simulink model "ModeloSimulador"  (R2020a)
settings: Solver=ode5  StartTime=0.0  StopTime=10.0  FixedStep=0.0001  RelTol=1e-3
values from neighbouring files (symbols this model uses):
  Bm = 0.008    [definirParametros.m]    (also in definirParametrosMotorElectroCraftDP300.m; definirParametrosMotorElectroCraftDPP728V120.m = Jm/tm; definirParametrosMotorElectroCraftDPP728V120_Optimizador.m = Jm/tm; definirParametrosMotorElectroCraftDPP728V120_v2.m = Jm/tm)
  dm = 0.3    [definirParametros.m]    (also in definirParametrosMotorElectroCraftDP300.m; definirParametrosMotorElectroCraftDPP728V120.m; definirParametrosMotorElectroCraftDPP728V120_Optimizador.m = 0.550061; definirParametrosMotorElectroCraftDPP728V120_v2.m = 0.550061)
  dmc = 0.5    [definirParametros.m]    (also in definirParametrosMotorElectroCraftDP300.m; definirParametrosMotorElectroCraftDPP728V120.m; definirParametrosMotorElectroCraftDPP728V120_Optimizador.m = 1.06911; definirParametrosMotorElectroCraftDPP728V120_v2.m = 1.06911)
  g = 9.8    [definirParametros.m]    (also in definirParametrosMotorElectroCraftDP300.m; definirParametrosMotorElectroCraftDPP728V120.m; definirParametrosMotorElectroCraftDPP728V120_Optimizador.m; definirParametrosMotorElectroCraftDPP728V120_v2.m)
  Jm = gramsCM2ToKgMeters2(12358.5)    [definirParametrosMotorElectroCraftDPP728V120.m]    (also in definirParametrosMotorElectroCraftDPP728V120_Optimizador.m; definirParametrosMotorElectroCraftDPP728V120_v2.m; definirParametrosMotorElectroCraftDPP728V120_v3.m; definirParametrosMotorElectroCraftRP34M221V90.m = gramsCM2ToKgMeters2(2718.9))
  Kb = 0.6    [definirParametros.m]    (also in definirParametrosMotorElectroCraftDP300.m = VoltagePerKRPMToVoltagePerHertz(12.3); definirParametrosMotorElectroCraftDPP728V120.m = VoltagePerKRPMToVoltagePerRadS(64.9); definirParametrosMotorElectroCraftDPP728V120_Optimizador.m = VoltagePerKRPMToVoltagePerRadS(64.9); definirParametrosMotorElectroCraftDPP728V120_v2.m = VoltagePerKRPMToVoltagePerRadS(64.9))
  Kt = 0.7274    [definirParametros.m]    (also in definirParametrosMotorElectroCraftDP300.m = newtonCMToNewtonM(11.722); definirParametrosMotorElectroCraftDPP728V120.m = newtonCMToNewtonM(62); definirParametrosMotorElectroCraftDPP728V120_Optimizador.m = newtonCMToNewtonM(62); definirParametrosMotorElectroCraftDPP728V120_v2.m = newtonCMToNewtonM(62))
  Lm = 4.3/1000    (= 0.0043)    [definirParametrosMotorElectroCraftDPP728V120.m]    (also in definirParametrosMotorElectroCraftDPP728V120_Optimizador.m; definirParametrosMotorElectroCraftDPP728V120_v2.m; definirParametrosMotorElectroCraftDPP728V120_v3.m; definirParametrosMotorElectroCraftDPP728V60.m = 0.0015)
  Mc = 200    [definirParametros.m]    (also in definirParametrosMotorElectroCraftDP300.m; definirParametrosMotorElectroCraftDPP728V120.m; definirParametrosMotorElectroCraftDPP728V120_Optimizador.m = 144.6; definirParametrosMotorElectroCraftDPP728V120_v2.m = 144.6)
  Mm = 100    [definirParametros.m]    (also in definirParametrosMotorElectroCraftDP300.m; definirParametrosMotorElectroCraftDPP728V120.m; definirParametrosMotorElectroCraftDPP728V120_Optimizador.m = 18.911; definirParametrosMotorElectroCraftDPP728V120_v2.m = 18.911)
  relacionEngranajes = 100.0/1    (= 100)    [definirParametros.m]    (also in definirParametrosMotorElectroCraftDP300.m = 1; definirParametrosMotorElectroCraftDPP728V120.m; definirParametrosMotorElectroCraftDPP728V120_Optimizador.m; definirParametrosMotorElectroCraftDPP728V120_v2.m)
  Rm = 1.55    [definirParametrosMotorElectroCraftDPP728V120.m]    (also in definirParametrosMotorElectroCraftDPP728V120_Optimizador.m; definirParametrosMotorElectroCraftDPP728V120_v2.m; definirParametrosMotorElectroCraftDPP728V120_v3.m; definirParametrosMotorElectroCraftDPP728V60.m = 0.72)
libraries: simulink x3
settings Model: Creator=rghuertaspaiva  LastModifiedBy=rghuertaspaiva

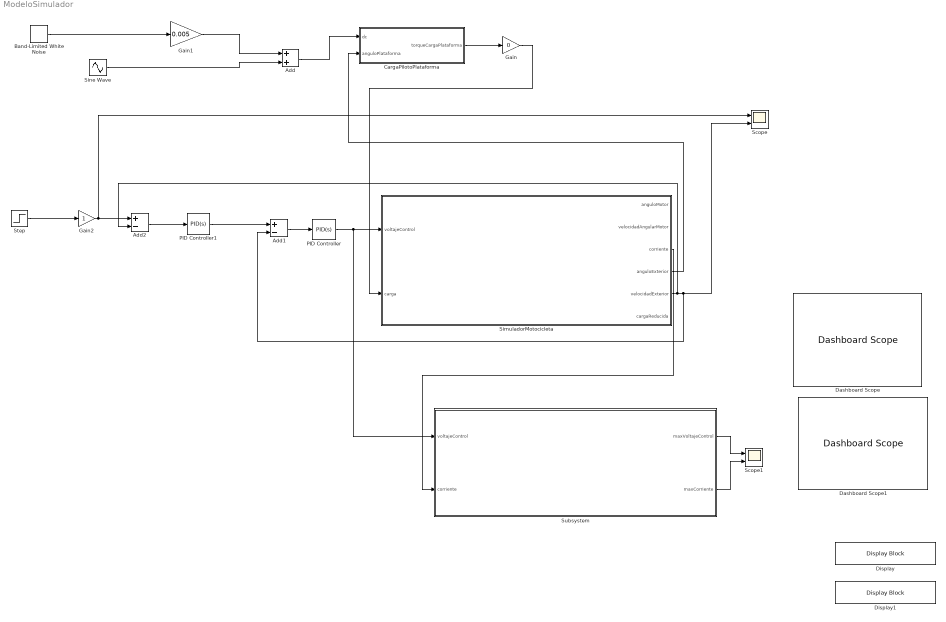
== system ModeloSimulador ==
  Add : Sum
  Add1 : Sum  Inputs=+-
  Add2 : Sum  Inputs=+-
  Band-Limited White Noise : simulink/Sources/Band-Limited White Noise  Cov=[.1]  Ts=0.001  seed=[23341]
  CargaPilotoPlataforma : Subsystem
  Dashboard Scope : DashboardScope
  Dashboard Scope1 : DashboardScope
  Display : DisplayBlock  LabelPosition=Hide  Format=short  Transparency=1
  Display1 : DisplayBlock  LabelPosition=Hide  Format=short  Transparency=1
  Gain : Gain  Gain=0
  Gain1 : Gain  Gain=0.005
  Gain2 : Gain
  PID Controller : simulink/Continuous/PID Controller  Controller=PID  Form=Parallel  TimeDomain=Continuous-time  UseExternalTs=off  SampleTime=-1  IntegratorMethod=Forward Euler  FilterMethod=Forward Euler  ControllerParametersSource=internal  P=0  I=825.13495714286  D=0  UseFilter=on  N=100  TunerSelectOption=Transfer Function Based (PID Tuner App)  InitialConditionSource=internal  InitialConditionForIntegrator=0  InitialConditionForFilter=0  DifferentiatorICPrevScaledInput=0  ExternalReset=none  TrackingMode=off  Kt=1  LimitOutput=off  UpperSaturationLimit=inf  LowerSaturationLimit=-inf  LinearizeAsGain=on  AntiWindupMode=none  Kb=1  POutMin=[]  POutMax=[]  IOutMin=[]  IOutMax=[]  DOutMin=[]  DOutMax=[]  NOutMin=[]  NOutMax=[]  SumOutMin=[]  SumOutMax=[]  SaturationOutMin=[]  SaturationOutMax=[]  PParamMin=[]  PParamMax=[]  IParamMin=[]  IParamMax=[]  DParamMin=[]  DParamMax=[]  NParamMin=[]  NParamMax=[]  KbParamMin=[]  KbParamMax=[]  KtParamMin=[]  KtParamMax=[]  KbOutMin=[]  KbOutMax=[]  KtOutMin=[]  KtOutMax=[]  IntegratorOutMin=[]  IntegratorOutMax=[]  FilterOutMin=[]  FilterOutMax=[]  SumI1OutMin=[]  SumI1OutMax=[]  SumI2OutMin=[]  SumI2OutMax=[]  SumI3OutMin=[]  SumI3OutMax=[]  SumI4OutMin=[]  SumI4OutMax=[]  SumDOutMin=[]  SumDOutMax=[]  DifferentiatorOutMin=[]  DifferentiatorOutMax=[]  FilterDiffOutCoefMin=[]  FilterDiffOutCoefMax=[]  ReciprocalOutMin=[]  ReciprocalOutMax=[]  SumDenOutMin=[]  SumDenOutMax=[]  SumNumOutMin=[]  SumNumOutMax=[]  DivideOutMin=[]  DivideOutMax=[]  UdiffTsProdOutMin=[]  UdiffTsProdOutMax=[]  NTsProdOutMin=[]  NTsProdOutMax=[]  UintegralTsProdOutMin=[]  UintegralTsProdOutMax=[]  UngainTsProdOutMin=[]  UngainTsProdOutMax=[]  IntegratorContinuousStateAttributes=''  IntegratorStateMustResolveToSignalObject=off  IntegratorRTWStateStorageClass=Auto  FilterContinuousStateAttributes=''  FilterStateMustResolveToSignalObject=off  FilterRTWStateStorageClass=Auto  ParallelPVariant=InternalParameters  IdealPVariant=Disabled  IVariant=InternalParameters  DVariant=InternalParameters  IntegratorVariant=Continuous  SatVariant=Disabled  AWVariant=Passthrough  PCopyVariant=Disabled  TRVariant=Disabled  FdbkBlocksVariant=Forward  IdealPFdbkVariant=Disabled  SatFdbkVariant=Disabled  DerivativeFilterVariant=ContFilter  NVariant=InternalParameters  NCopyVariant=Disabled  FilterICVariant=InternalICsFilter  IntegratorICVariant=InternalICs  ExternalResetVariant=Disabled  TRSumVariant=Passthrough  SumFdbkVariant=Disabled  SumVariant=Sum_PID  TsampFilterVariant=InternalTs  TsampNgainVariant=Passthrough  TsampIntegralVariant=Passthrough
  PID Controller1 : simulink/Continuous/PID Controller  Controller=PID  Form=Parallel  TimeDomain=Continuous-time  UseExternalTs=off  SampleTime=-1  IntegratorMethod=Forward Euler  FilterMethod=Forward Euler  ControllerParametersSource=internal  P=0  I=2.1974250640263  D=0  UseFilter=on  N=100  TunerSelectOption=Transfer Function Based (PID Tuner App)  InitialConditionSource=internal  InitialConditionForIntegrator=0  InitialConditionForFilter=0  DifferentiatorICPrevScaledInput=0  ExternalReset=none  TrackingMode=off  Kt=1  LimitOutput=off  UpperSaturationLimit=inf  LowerSaturationLimit=-inf  LinearizeAsGain=on  AntiWindupMode=none  Kb=1  POutMin=[]  POutMax=[]  IOutMin=[]  IOutMax=[]  DOutMin=[]  DOutMax=[]  NOutMin=[]  NOutMax=[]  SumOutMin=[]  SumOutMax=[]  SaturationOutMin=[]  SaturationOutMax=[]  PParamMin=[]  PParamMax=[]  IParamMin=[]  IParamMax=[]  DParamMin=[]  DParamMax=[]  NParamMin=[]  NParamMax=[]  KbParamMin=[]  KbParamMax=[]  KtParamMin=[]  KtParamMax=[]  KbOutMin=[]  KbOutMax=[]  KtOutMin=[]  KtOutMax=[]  IntegratorOutMin=[]  IntegratorOutMax=[]  FilterOutMin=[]  FilterOutMax=[]  SumI1OutMin=[]  SumI1OutMax=[]  SumI2OutMin=[]  SumI2OutMax=[]  SumI3OutMin=[]  SumI3OutMax=[]  SumI4OutMin=[]  SumI4OutMax=[]  SumDOutMin=[]  SumDOutMax=[]  DifferentiatorOutMin=[]  DifferentiatorOutMax=[]  FilterDiffOutCoefMin=[]  FilterDiffOutCoefMax=[]  ReciprocalOutMin=[]  ReciprocalOutMax=[]  SumDenOutMin=[]  SumDenOutMax=[]  SumNumOutMin=[]  SumNumOutMax=[]  DivideOutMin=[]  DivideOutMax=[]  UdiffTsProdOutMin=[]  UdiffTsProdOutMax=[]  NTsProdOutMin=[]  NTsProdOutMax=[]  UintegralTsProdOutMin=[]  UintegralTsProdOutMax=[]  UngainTsProdOutMin=[]  UngainTsProdOutMax=[]  IntegratorContinuousStateAttributes=''  IntegratorStateMustResolveToSignalObject=off  IntegratorRTWStateStorageClass=Auto  FilterContinuousStateAttributes=''  FilterStateMustResolveToSignalObject=off  FilterRTWStateStorageClass=Auto  ParallelPVariant=InternalParameters  IdealPVariant=Disabled  IVariant=InternalParameters  DVariant=InternalParameters  IntegratorVariant=Continuous  SatVariant=Disabled  AWVariant=Passthrough  PCopyVariant=Disabled  TRVariant=Disabled  FdbkBlocksVariant=Forward  IdealPFdbkVariant=Disabled  SatFdbkVariant=Disabled  DerivativeFilterVariant=ContFilter  NVariant=InternalParameters  NCopyVariant=Disabled  FilterICVariant=InternalICsFilter  IntegratorICVariant=InternalICs  ExternalResetVariant=Disabled  TRSumVariant=Passthrough  SumFdbkVariant=Disabled  SumVariant=Sum_PID  TsampFilterVariant=InternalTs  TsampNgainVariant=Passthrough  TsampIntegralVariant=Passthrough
  Scope : Scope  NumInputPorts=2
  Scope1 : Scope  NumInputPorts=2
  SimuladorMotocicleta : Subsystem
  Sine Wave : Sin  Amplitude=0.015  SampleTime=0
  Step : Step  After=deg2rad(30)  SampleTime=0
  Subsystem : Subsystem
  wires:
  Gain/1 -> SimuladorMotocicleta/2(carga)
  Gain1/1 -> Add/1
  Sine Wave/1 -> Add/2
  Add/1 -> CargaPilotoPlataforma/1(dc)
  SimuladorMotocicleta/4(anguloExterior) -> CargaPilotoPlataforma/2(anguloPlataforma)
  CargaPilotoPlataforma/1(torqueCargaPlataforma) -> Gain/1
  Band-Limited White Noise/1 -> Gain1/1
  PID Controller/1 -> Subsystem/1(voltajeControl), SimuladorMotocicleta/1(voltajeControl)
  Add1/1 -> PID Controller/1
  Step/1 -> Gain2/1
  SimuladorMotocicleta/5(velocidadExterior) -> Scope/2, Add1/2, Add2/2
  Gain2/1 -> Scope/1, Add2/1
  PID Controller1/1 -> Add1/1
  Add2/1 -> PID Controller1/1
  SimuladorMotocicleta/3(corriente) -> Subsystem/2(corriente)
  Subsystem/1(maxVoltajeControl) -> Scope1/1
  Subsystem/2(maxCorriente) -> Scope1/2

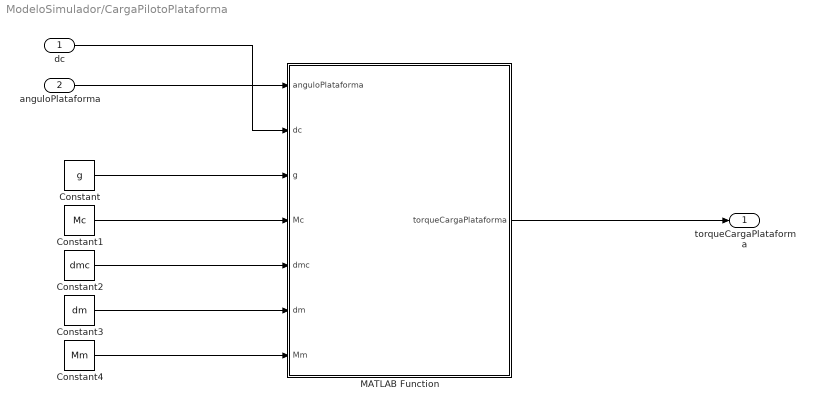
== system ModeloSimulador/CargaPilotoPlataforma ==
  dc : Inport
  anguloPlataforma : Inport  Port=2
  Constant : Constant  Value=g
  Constant1 : Constant  Value=Mc
  Constant2 : Constant  Value=dmc
  Constant3 : Constant  Value=dm
  Constant4 : Constant  Value=Mm
  MATLAB Function : MATLAB Function  TreatAsAtomicUnit=on
  torqueCargaPlataforma : Outport
  wires:
  dc/1 -> MATLAB Function/2(dc)
  anguloPlataforma/1 -> MATLAB Function/1(anguloPlataforma)
  Constant/1 -> MATLAB Function/3(g)
  Constant1/1 -> MATLAB Function/4(Mc)
  Constant2/1 -> MATLAB Function/5(dmc)
  Constant3/1 -> MATLAB Function/6(dm)
  Constant4/1 -> MATLAB Function/7(Mm)
  MATLAB Function/1(torqueCargaPlataforma) -> torqueCargaPlataforma/1

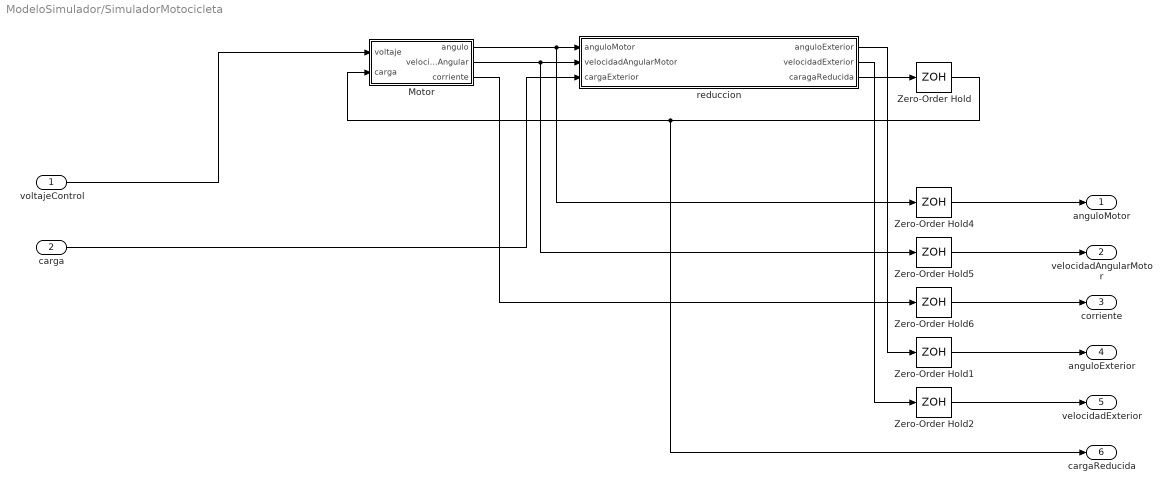
== system ModeloSimulador/SimuladorMotocicleta ==
  voltajeControl : Inport
  carga : Inport  Port=2
  Motor : Subsystem
  Zero-Order Hold{,1..2,4..6} (6 alike) : ZeroOrderHold  SampleTime=-1
  reduccion : Subsystem
  anguloMotor : Outport
  velocidadAngularMotor : Outport  Port=2
  corriente : Outport  Port=3
  anguloExterior : Outport  Port=4
  velocidadExterior : Outport  Port=5
  cargaReducida : Outport  Port=6
  wires:
  voltajeControl/1 -> Motor/1(voltaje)
  Motor/1(angulo) -> Zero-Order Hold4/1, reduccion/1(anguloMotor)
  Motor/2(velocidadAngular) -> Zero-Order Hold5/1, reduccion/2(velocidadAngularMotor)
  carga/1 -> reduccion/3(cargaExterior)
  reduccion/3(caragaReducida) -> Zero-Order Hold/1
  Motor/3(corriente) -> Zero-Order Hold6/1
  reduccion/1(anguloExterior) -> Zero-Order Hold1/1
  reduccion/2(velocidadExterior) -> Zero-Order Hold2/1
  Zero-Order Hold1/1 -> anguloExterior/1
  Zero-Order Hold2/1 -> velocidadExterior/1
  Zero-Order Hold/1 -> cargaReducida/1, Motor/2(carga)
  Zero-Order Hold4/1 -> anguloMotor/1
  Zero-Order Hold5/1 -> velocidadAngularMotor/1
  Zero-Order Hold6/1 -> corriente/1

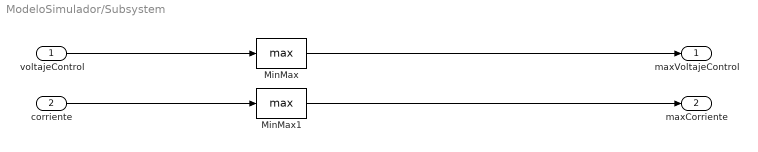
== system ModeloSimulador/Subsystem ==
  voltajeControl : Inport
  corriente : Inport  Port=2
  MinMax : MinMax  Function=max
  MinMax1 : MinMax  Function=max
  maxVoltajeControl : Outport
  maxCorriente : Outport  Port=2
  wires:
  MinMax/1 -> maxVoltajeControl/1
  voltajeControl/1 -> MinMax/1
  corriente/1 -> MinMax1/1
  MinMax1/1 -> maxCorriente/1

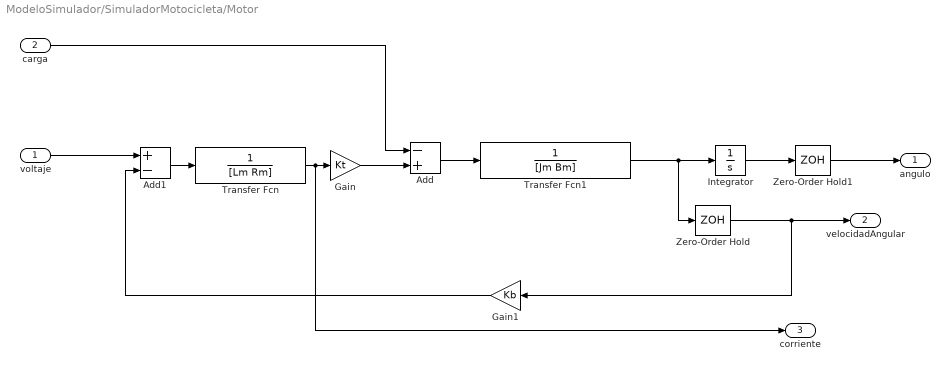
== system ModeloSimulador/SimuladorMotocicleta/Motor ==
  voltaje : Inport
  carga : Inport  Port=2
  Add : Sum  Inputs=-+
  Add1 : Sum  Inputs=+-
  Gain : Gain  Gain=Kt
  Gain1 : Gain  Gain=Kb
  Integrator : Integrator
  Transfer Fcn : TransferFcn  Denominator=[Lm Rm]
  Transfer Fcn1 : TransferFcn  Denominator=[Jm Bm]
  Zero-Order Hold : ZeroOrderHold  SampleTime=-1
  Zero-Order Hold1 : ZeroOrderHold  SampleTime=-1
  angulo : Outport
  velocidadAngular : Outport  Port=2
  corriente : Outport  Port=3
  wires:
  Gain/1 -> Add/2
  Add/1 -> Transfer Fcn1/1
  Transfer Fcn/1 -> corriente/1, Gain/1
  Transfer Fcn1/1 -> Integrator/1, Zero-Order Hold/1
  Zero-Order Hold/1 -> Gain1/1, velocidadAngular/1
  Integrator/1 -> Zero-Order Hold1/1
  voltaje/1 -> Add1/1
  Add1/1 -> Transfer Fcn/1
  Gain1/1 -> Add1/2
  carga/1 -> Add/1
  Zero-Order Hold1/1 -> angulo/1

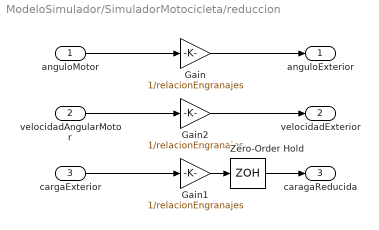
== system ModeloSimulador/SimuladorMotocicleta/reduccion ==
  anguloMotor : Inport
  velocidadAngularMotor : Inport  Port=2
  cargaExterior : Inport  Port=3
  Gain : Gain  Gain=1/relacionEngranajes
  Gain1 : Gain  Gain=1/relacionEngranajes
  Gain2 : Gain  Gain=1/relacionEngranajes
  Zero-Order Hold : ZeroOrderHold  SampleTime=-1
  anguloExterior : Outport
  velocidadExterior : Outport  Port=2
  caragaReducida : Outport  Port=3
  wires:
  anguloMotor/1 -> Gain/1
  Gain/1 -> anguloExterior/1
  cargaExterior/1 -> Gain1/1
  Gain1/1 -> Zero-Order Hold/1
  velocidadAngularMotor/1 -> Gain2/1
  Gain2/1 -> velocidadExterior/1
  Zero-Order Hold/1 -> caragaReducida/1

== matlab function ModeloSimulador/CargaPilotoPlataforma/MATLAB Function ==
  data: anguloPlataforma input; torqueCargaPlataforma output; dc input; g input; Mc input; dmc input; dm input; Mm input
function torqueCargaPlataforma = torquePlataformaPiloto(anguloPlataforma, dc, g, Mc, dmc, dm, Mm)

%torqueCargaPlataforma = 0;
% torqueCargaPlataforma = g*( dc*Mc*cos(anguloPlataforma) + ...
%                             (dmc*Mc + dm*(Mc + Mm))*sin(anguloPlataforma) ...
%                           );
torqueCargaPlataforma =  g*( 0*Mc*cos(anguloPlataforma) + ...
                             (dmc*Mc + dm*(Mc + Mm))*sin(anguloPlataforma) ...
                           );
%t=0;
